simulink model "vehicle"  (R2024b)
settings: Solver=ode23s  StartTime=0.0  StopTime=t_f  FixedStep=1e-4  RelTol=1e-5
undefined symbols (not defined in the file): Earth, front_steer, front_torque, grav, rear_steer, rear_torque, steer_time, torque_time, vehicle_mass, WGS84
libraries: aerolib6dof2 x1
settings Model: VariantFading=off  Creator=yevge  LastModifiedBy=yevge
settings SolverCC: ZcThreshold=1e-5  ZeroCrossControl=DisableAll  ZeroCrossAlgorithm=Adaptive
settings RTWCC: CheckMdlBeforeBuild=Error

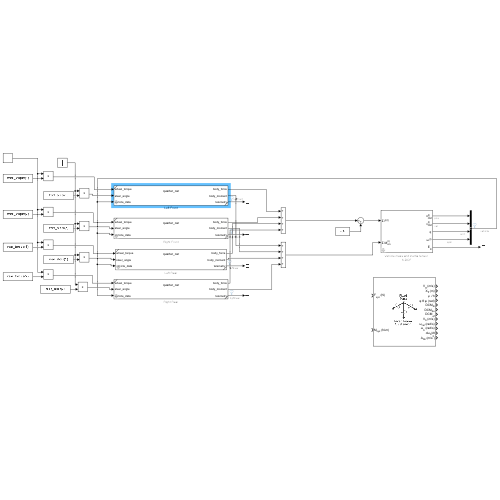
[thumbnail: Simulink's stored preview of the top-level diagram]
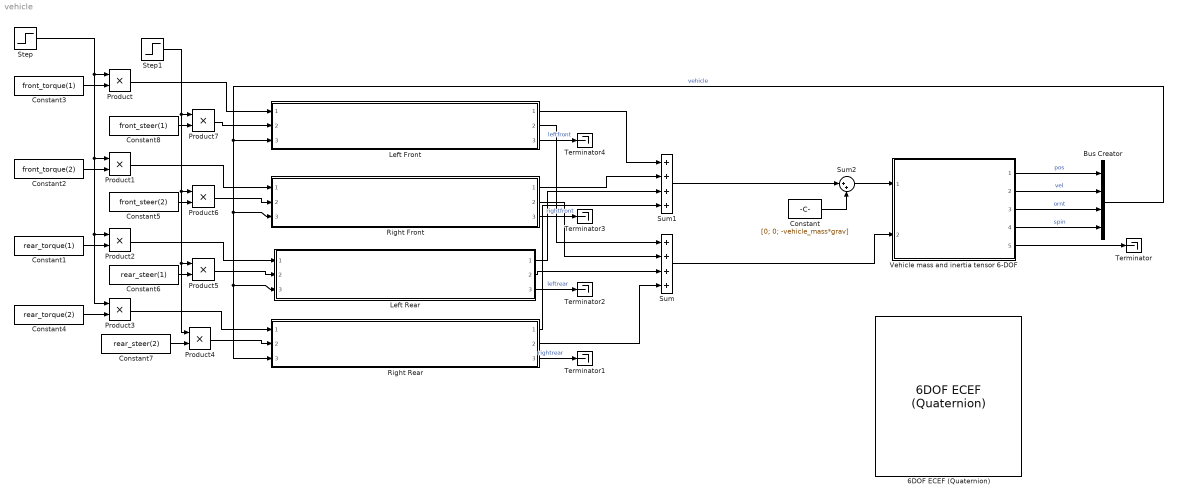
== system vehicle ==
  6DOF ECEF (Quaternion) : aerolib6dof2/6DOF ECEF (Quaternion)  units=Metric (MKS)  mtype=Fixed  xg_0=[0 0 0]  Vm_0=[0 0 0]  eul_0=[0 0 0]  pm_0=[0 0 0]  mass_0=1.0  mass_e=0.5  mass_f=2.0  inertia=eye(3)  inertia_e=eye(3)  inertia_f=2*eye(3)  vre_flag=on  abi_flag=off  ptype=Earth (WGS84)  R=6378137  F=1/298.257223563  w_E=7292115e-11  angle_in=Internal  LPM0=0  quat_statename=''  pm_statename=''  Vm_statename=''  posfixedframe_statename=''  posinertial_statename=''  LPM_statename=''  mass_statename=''
  Bus Creator : BusCreator  Inputs=4
  Constant : Constant  Value=[0; 0; -vehicle_mass*grav]
  Constant1 : Constant  Value=rear_torque(1)
  Constant2 : Constant  Value=front_torque(2)
  Constant3 : Constant  Value=front_torque(1)
  Constant4 : Constant  Value=rear_torque(2)
  Constant5 : Constant  Value=front_steer(2)
  Constant6 : Constant  Value=rear_steer(1)
  Constant7 : Constant  Value=rear_steer(2)
  Constant8 : Constant  Value=front_steer(1)
  Left Front : Subsystem  ReferencedSubsystem=quarter_car  radius=wheel_radius  spin_inertia=wheel_inertia  offset=patch_leftfront  ride_rate=front_stiffness  damp_rate=front_damping  C_i=NaN  C_a=NaN  min_velocity=min_velocity  initial_spin=0
  Left Rear : Subsystem  ReferencedSubsystem=quarter_car  radius=wheel_radius  spin_inertia=wheel_inertia  offset=patch_leftrear  ride_rate=rear_stiffness  damp_rate=rear_damping  C_i=NaN  C_a=NaN  min_velocity=1e-3  initial_spin=0
  Product{,1..7} (8 alike) : Product
  Right Front : Subsystem  ReferencedSubsystem=quarter_car  radius=wheel_radius  spin_inertia=wheel_inertia  offset=patch_rightfront  ride_rate=front_stiffness  damp_rate=front_damping  C_i=NaN  C_a=NaN  min_velocity=1e-3  initial_spin=0
  Right Rear : Subsystem  ReferencedSubsystem=quarter_car  radius=wheel_radius  spin_inertia=wheel_inertia  offset=patch_rightrear  ride_rate=rear_stiffness  damp_rate=rear_damping  C_i=NaN  C_a=NaN  min_velocity=1e-3  initial_spin=0
  Step : Step  Time=torque_time  SampleTime=0
  Step1 : Step  Time=steer_time  SampleTime=0
  Sum : Sum  Inputs=++++
  Sum1 : Sum  Inputs=++++
  Sum2 : Sum  Inputs=|++
  Terminator{,1..4} (5 alike) : Terminator
  Vehicle mass and inertia tensor 6-DOF : Subsystem  ReferencedSubsystem=rigid_body_sixdof  pos_0=vehicle_pos_0  vel_0=vehicle_vel_0  ornt_0=vehicle_ornt_0  mass=vehicle_mass  inertia=vehicle_inertia  spin_0=vehicle_spin_0
  wires:
  Constant/1 -> Sum2/2
  Vehicle mass and inertia tensor 6-DOF/2 -> Bus Creator/2  "vel"
  Vehicle mass and inertia tensor 6-DOF/4 -> Bus Creator/4  "spin"
  Sum1/1 -> Sum2/1
  Sum/1 -> Vehicle mass and inertia tensor 6-DOF/2
  Sum2/1 -> Vehicle mass and inertia tensor 6-DOF/1
  Vehicle mass and inertia tensor 6-DOF/5 -> Terminator/1
  Left Front/1 -> Sum1/1
  Right Front/1 -> Sum1/2
  Left Rear/1 -> Sum1/3
  Right Rear/1 -> Sum1/4
  Right Rear/2 -> Sum/4
  Left Rear/2 -> Sum/3
  Right Front/2 -> Sum/2
  Left Front/2 -> Sum/1
  Vehicle mass and inertia tensor 6-DOF/1 -> Bus Creator/1  "pos"
  Bus Creator/1 -> Right Rear/3, Left Rear/3, Right Front/3, Left Front/3  "vehicle"
  Right Rear/3 -> Terminator1/1  "rightrear"
  Left Rear/3 -> Terminator2/1  "leftrear"
  Right Front/3 -> Terminator3/1  "rightfront"
  Left Front/3 -> Terminator4/1  "leftfront"
  Vehicle mass and inertia tensor 6-DOF/3 -> Bus Creator/3  "ornt"
  Constant3/1 -> Product/2
  Constant2/1 -> Product1/2
  Constant1/1 -> Product2/2
  Constant4/1 -> Product3/2
  Product3/1 -> Right Rear/1
  Product2/1 -> Left Rear/1
  Product1/1 -> Right Front/1
  Product/1 -> Left Front/1
  Product4/1 -> Right Rear/2
  Constant7/1 -> Product4/2
  Constant6/1 -> Product5/2
  Constant5/1 -> Product6/2
  Constant8/1 -> Product7/2
  Product7/1 -> Left Front/2
  Product6/1 -> Right Front/2
  Product5/1 -> Left Rear/2
  Step/1 -> Product3/1, Product2/1, Product1/1, Product/1
  Step1/1 -> Product4/1, Product5/1, Product6/1, Product7/1
